simulink subsystem "Long_Vert_Aero_Forces_Moments1"  (R2025b)
settings: Solver=VariableStepAuto  StartTime=0.0  StopTime=10.0  RelTol=1e-3
values from neighbouring files (symbols this model uses):
  Sref = 4702    [Sim6DOF_Init.m]
undefined symbols (not defined in the file or in its folder): Cbar, CD1, CD_alpha, CD_delEle, CD_ih, CL1, CL_alpha, CL_delEle, CL_ih, CM_0, CM_alpha, CM_delEle, CM_ih
libraries: simulink_extras x3
settings Model: Creator=cdriggs  LastModifiedBy=samuelvelasquez

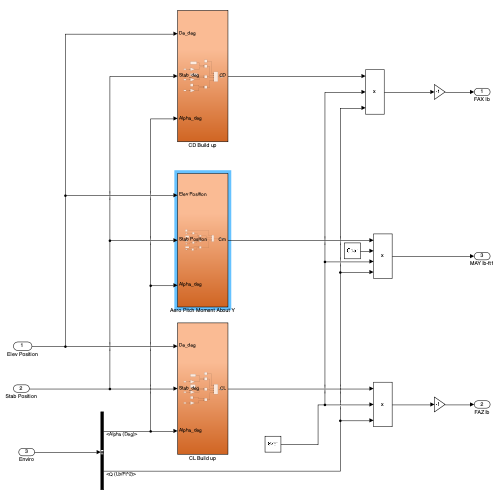
[thumbnail: Simulink's stored preview of the top-level diagram]
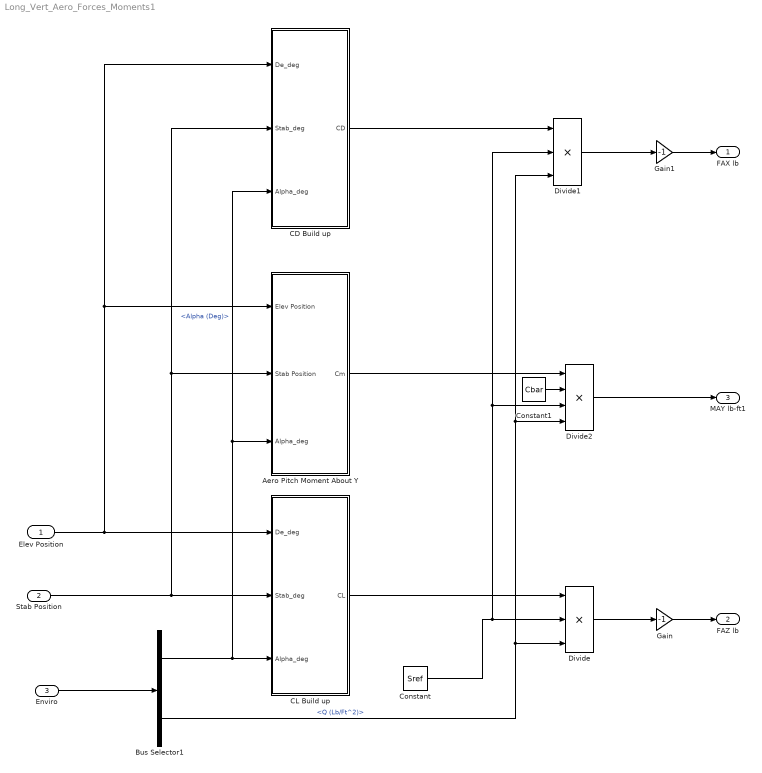
== system Long_Vert_Aero_Forces_Moments1 ==
  Elev Position : Inport
  Stab Position : Inport  Port=2
  Enviro : Inport  Port=3
  Aero Pitch Moment About Y : Subsystem
  Bus Selector1 : BusSelector  OutputSignals=Alpha (Deg),Q (Lb/Ft^2)
  CD Build up : Subsystem
  CL Build up : Subsystem
  Constant : Constant  Value=Sref
  Constant1 : Constant  Value=Cbar
  Divide : Product  Inputs=***
  Divide1 : Product  Inputs=***
  Divide2 : Product  Inputs=****
  Gain : Gain  Gain=-1
  Gain1 : Gain  Gain=-1
  FAX lb : Outport
  FAZ lb : Outport  Port=2
  MAY lb-ft1 : Outport  Port=3
  wires:
  CL Build up/1(CL) -> Divide/1
  Enviro/1 -> Bus Selector1/1
  CD Build up/1(CD) -> Divide1/1
  Gain/1 -> FAZ lb/1
  Constant/1 -> Divide1/2, Divide2/3, Divide/2
  Bus Selector1/2 -> Divide/3, Divide2/4, Divide1/3  "<Q (Lb/Ft^2)>"
  Gain1/1 -> FAX lb/1
  Stab Position/1 -> CL Build up/2(Stab_deg), Aero Pitch Moment About Y/2(Stab Position), CD Build up/2(Stab_deg)
  Divide/1 -> Gain/1
  Divide1/1 -> Gain1/1
  Elev Position/1 -> Aero Pitch Moment About Y/1(Elev Position), CD Build up/1(De_deg), CL Build up/1(De_deg)
  Bus Selector1/1 -> Aero Pitch Moment About Y/3(Alpha_deg), CD Build up/3(Alpha_deg), CL Build up/3(Alpha_deg)  "<Alpha (Deg)>"
  Aero Pitch Moment About Y/1(Cm) -> Divide2/1
  Constant1/1 -> Divide2/2
  Divide2/1 -> MAY lb-ft1/1

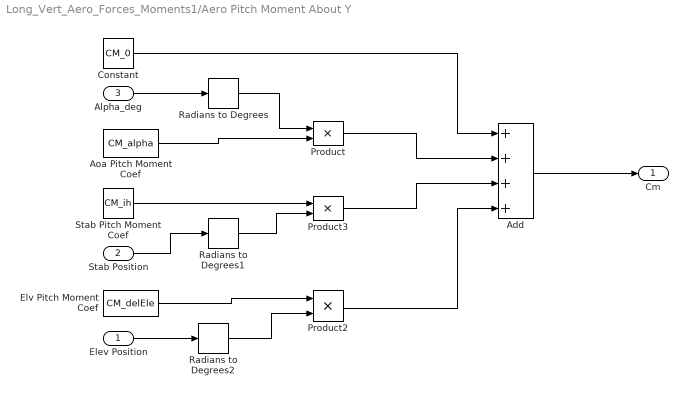
== system Long_Vert_Aero_Forces_Moments1/Aero Pitch Moment About Y ==
  Elev Position : Inport
  Stab Position : Inport  Port=2
  Alpha_deg : Inport  Port=3
  Add : Sum  Inputs=++++
  Aoa Pitch Moment Coef : Constant  Value=CM_alpha
  Constant : Constant  Value=CM_0
  Elv Pitch Moment Coef : Constant  Value=CM_delEle
  Product : Product
  Product2 : Product
  Product3 : Product
  Radians to Degrees : simulink_extras/Transformations/Radians to Degrees
  Radians to Degrees1 : simulink_extras/Transformations/Radians to Degrees
  Radians to Degrees2 : simulink_extras/Transformations/Radians to Degrees
  Stab Pitch Moment Coef : Constant  Value=CM_ih
  Cm : Outport
  wires:
  Stab Position/1 -> Radians to Degrees1/1
  Alpha_deg/1 -> Radians to Degrees/1
  Aoa Pitch Moment Coef/1 -> Product/2
  Stab Pitch Moment Coef/1 -> Product3/1
  Elv Pitch Moment Coef/1 -> Product2/1
  Elev Position/1 -> Radians to Degrees2/1
  Radians to Degrees2/1 -> Product2/2
  Radians to Degrees1/1 -> Product3/2
  Product3/1 -> Add/3
  Radians to Degrees/1 -> Product/1
  Add/1 -> Cm/1
  Product2/1 -> Add/4
  Product/1 -> Add/2
  Constant/1 -> Add/1

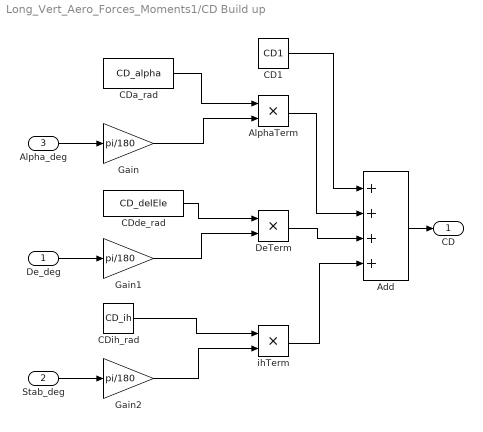
== system Long_Vert_Aero_Forces_Moments1/CD Build up ==
  De_deg : Inport
  Stab_deg : Inport  Port=2
  Alpha_deg : Inport  Port=3
  Add : Sum  Inputs=++++
  AlphaTerm : Product
  CD1 : Constant  Value=CD1
  CDa_rad : Constant  Value=CD_alpha
  CDde_rad : Constant  Value=CD_delEle
  CDih_rad : Constant  Value=CD_ih
  DeTerm : Product
  Gain : Gain  Gain=pi/180
  Gain1 : Gain  Gain=pi/180
  Gain2 : Gain  Gain=pi/180
  ihTerm : Product
  CD : Outport
  wires:
  CD1/1 -> Add/1
  AlphaTerm/1 -> Add/2
  DeTerm/1 -> Add/3
  ihTerm/1 -> Add/4
  Add/1 -> CD/1
  Gain2/1 -> ihTerm/2
  CDih_rad/1 -> ihTerm/1
  CDde_rad/1 -> DeTerm/1
  Gain1/1 -> DeTerm/2
  CDa_rad/1 -> AlphaTerm/1
  Gain/1 -> AlphaTerm/2
  De_deg/1 -> Gain1/1
  Stab_deg/1 -> Gain2/1
  Alpha_deg/1 -> Gain/1

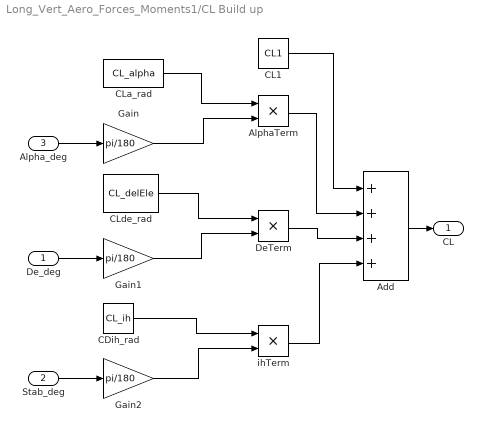
== system Long_Vert_Aero_Forces_Moments1/CL Build up ==
  De_deg : Inport
  Stab_deg : Inport  Port=2
  Alpha_deg : Inport  Port=3
  Add : Sum  Inputs=++++
  AlphaTerm : Product
  CDih_rad : Constant  Value=CL_ih
  CL1 : Constant  Value=CL1
  CLa_rad : Constant  Value=CL_alpha
  CLde_rad : Constant  Value=CL_delEle
  DeTerm : Product
  Gain : Gain  Gain=pi/180
  Gain1 : Gain  Gain=pi/180
  Gain2 : Gain  Gain=pi/180
  ihTerm : Product
  CL : Outport
  wires:
  CL1/1 -> Add/1
  AlphaTerm/1 -> Add/2
  DeTerm/1 -> Add/3
  ihTerm/1 -> Add/4
  Add/1 -> CL/1
  Gain2/1 -> ihTerm/2
  CDih_rad/1 -> ihTerm/1
  CLde_rad/1 -> DeTerm/1
  Gain1/1 -> DeTerm/2
  CLa_rad/1 -> AlphaTerm/1
  Gain/1 -> AlphaTerm/2
  De_deg/1 -> Gain1/1
  Stab_deg/1 -> Gain2/1
  Alpha_deg/1 -> Gain/1
